simulink model "RTP_V5_Regelung_DKL_Test_P_Regler_Modell_2018a"  (R2020a)
settings: Solver=ode45  StartTime=0.0  StopTime=2  MaxStep=1e-3  RelTol=1e-3  EnableMultiTasking=on
values from neighbouring files (symbols this model uses):
  G_M = cphi    (= 0.03)    [RTP_V5_Regelung_DKL_Test_PIDT1_Regler.m]    (also in RTP_V5_Regelung_DKL_Test_P_Regler.m)
  G_Rueck = cphi    (= 0.03)    [RTP_V5_Regelung_DKL_Test_PIDT1_Regler.m]    (also in RTP_V5_Regelung_DKL_Test_P_Regler.m)
  K = 0.0508    [RTP_V5_Regelung_DKL_Test_PIDT1_Regler.m]    (also in RTP_V5_Regelung_DKL_Test_P_Regler.m = 0.0509)
  n1 = [La/Ra, 1]    [RTP_V5_Regelung_DKL_Test_PIDT1_Regler.m]    (also in RTP_V5_Regelung_DKL_Test_P_Regler.m)
  n3 = [J, 0]    [RTP_V5_Regelung_DKL_Test_PIDT1_Regler.m]    (also in RTP_V5_Regelung_DKL_Test_P_Regler.m)
  n4 = pi    (= 3.14159265359)    [RTP_V5_Regelung_DKL_Test_PIDT1_Regler.m]    (also in RTP_V5_Regelung_DKL_Test_P_Regler.m = 20)
  sat = 1    [RTP_V5_Regelung_DKL_Test_PIDT1_Regler.m]    (also in RTP_V5_Regelung_DKL_Test_P_Regler.m)
  T = 0.004    [RTP_V5_Regelung_DKL_Test_PIDT1_Regler.m]    (also in RTP_V5_Regelung_DKL_Test_P_Regler.m)
  Tn = Tz1 + Tz2 - T    (= 0.129333333333)    [RTP_V5_Regelung_DKL_Test_PIDT1_Regler.m]    (also in RTP_V5_Regelung_DKL_Test_P_Regler.m)
  Tv = Tz1*Tz2 / Tn - T    (= 0.0217731958763)    [RTP_V5_Regelung_DKL_Test_PIDT1_Regler.m]    (also in RTP_V5_Regelung_DKL_Test_P_Regler.m)
  U_mot = 12    [RTP_V5_Regelung_DKL_Test_PIDT1_Regler.m]    (also in RTP_V5_Regelung_DKL_Test_P_Regler.m)
  z1 = 1/Ra    (= 0.285714285714)    [RTP_V5_Regelung_DKL_Test_PIDT1_Regler.m]    (also in RTP_V5_Regelung_DKL_Test_P_Regler.m)
  z3 = 1    [RTP_V5_Regelung_DKL_Test_PIDT1_Regler.m]    (also in RTP_V5_Regelung_DKL_Test_P_Regler.m)
  z4 = i_Getr*180    (= 9)    [RTP_V5_Regelung_DKL_Test_PIDT1_Regler.m]    (also in RTP_V5_Regelung_DKL_Test_P_Regler.m = 57.2957795131)
settings Model: Creator=bruedig  LastModifiedBy=Admin
settings DataIOCC: LimitDataPoints=on  SaveFormat=Array  SignalLoggingSaveFormat=ModelDataLogs  ReturnWorkspaceOutputs=off
settings OptimizationCC: BooleanDataType=off  ExpressionDepthLimit=2147483647  InitFltsAndDblsToZero=on  LifeSpan=inf
settings DebuggingCC: SaveWithParameterizedLinksMsg=none  UnderspecifiedInitializationDetection=Classic  MergeDetectMultiDrivingBlocksExec=none  SignalResolutionControl=TryResolveAllWithWarning  MultiTaskDSMMsg=warning  MultiTaskCondExecSysMsg=none  FcnCallInpInsideContextMsg=warning  StateNameClashWarn=warning  SFUnexpectedBacktrackingDiag=warning  SFNoUnconditionalDefaultTransitionDiag=warning  SFExecutionAtInitializationDiag=none  ArithmeticOperatorsInVariantConditions=warning
settings HardwareCC: ProdBitPerPointer=32  ProdBitPerSizeT=32  ProdBitPerPtrDiffT=32  ProdLargestAtomicFloat=None  ProdIntDivRoundTo=Undefined  ProdEndianess=Unspecified  ProdWordSize=32  ProdHWDeviceType=32-bit Generic  TargetUnknown=on
settings ModelReferenceCC: PropagateSignalLabelsOutOfModel=off
settings SFSimCC: SimUseLocalCustomCode=off  CustomCodeUndefinedFunction=UseInterfaceOnly
settings RTWCC: RTWUseLocalCustomCode=off
settings CodeAppCC: StateflowObjectComments=on
settings GRTTargetCC: TargetFcnLib=ansi_tfl_tmw.mat  TargetLangStandard=C89/C90 (ANSI)  CombineOutputUpdateFcns=off  GRTInterface=on
settings ConfigComp: CovMetricSettings=dw  CovHtmlReporting=on  CovSaveCumulativeToWorkspaceVar=on  CovSaveSingleToWorkspaceVar=on  CovExternalEMLEnable=off

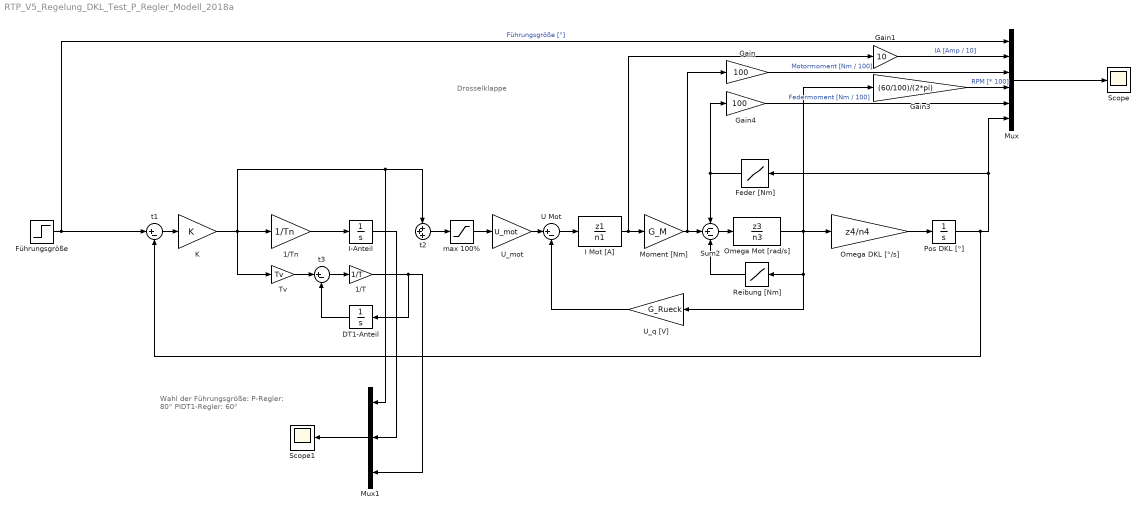
== system RTP_V5_Regelung_DKL_Test_P_Regler_Modell_2018a ==
  note: Wahl der Führungsgröße:
      | P-Regler: 80°
      | PIDT1-Regler: 60°
  note: Drosselklappe
  1/T : Gain  Gain=1/T  SaturateOnIntegerOverflow=on  OutDataTypeStr=Inherit: Same as input  ParamDataTypeStr=Inherit: Same as input
  1/Tn : Gain  Gain=1/Tn  SaturateOnIntegerOverflow=on  OutDataTypeStr=Inherit: Same as input  ParamDataTypeStr=Inherit: Same as input
  DT1-Anteil : Integrator
  Feder [Nm] : Lookup  InputValues="[-0.1,      0,         3.7,     3.8,     90,   90.1]"  Table="[-0.1,   -0.02450,   -0.02430,   0.02430,     0.02916,    0.1]"  SaturateOnIntegerOverflow=on
  Führungsgröße : Step  Time=0  Before=3.7  After=60  SampleTime=0
  Gain : Gain  Gain=100
  Gain1 : Gain  Gain=10
  Gain3 : Gain  Gain=(60/100)/(2*pi)  SaturateOnIntegerOverflow=on  OutDataTypeStr=Inherit: Same as input  ParamDataTypeStr=Inherit: Same as input
  Gain4 : Gain  Gain=100
  I Mot [A] : TransferFcn  Numerator=z1  Denominator=n1
  I-Anteil : Integrator  UpperSaturationLimit=1  LowerSaturationLimit=0
  K : Gain  Gain=K  SaturateOnIntegerOverflow=on  OutDataTypeStr=Inherit: Same as input  ParamDataTypeStr=Inherit: Same as input
  Moment [Nm] : Gain  Gain=G_M  SaturateOnIntegerOverflow=on  OutDataTypeStr=Inherit: Same as input  ParamDataTypeStr=Inherit: Same as input
  Mux : Mux  Inputs=6
  Mux1 : Mux  Inputs=3
  Omega DKL [°/s] : Gain  Gain=z4/n4  SaturateOnIntegerOverflow=on  OutDataTypeStr=Inherit: Same as input  ParamDataTypeStr=Inherit: Same as input
  Omega Mot [rad/s] : TransferFcn  Numerator=z3  Denominator=n3
  Pos DKL [°] : Integrator  InitialCondition=3.7
  Reibung [Nm] : Lookup  InputValues="[-1,              -0.01,           0.01,           1]"  Table="[-0.009,   -0.009,   0.009,   0.009]"  SaturateOnIntegerOverflow=on
  Scope : Scope
  Scope1 : Scope
  Sum2 : Sum  Inputs=-+-  InputSameDT=on  SaturateOnIntegerOverflow=on  OutDataTypeStr=Inherit: Same as first input
  Tv : Gain  Gain=Tv  SaturateOnIntegerOverflow=on  OutDataTypeStr=Inherit: Same as input  ParamDataTypeStr=Inherit: Same as input
  U Mot : Sum  Description=Motorspannung  Inputs=|+-  InputSameDT=on  SaturateOnIntegerOverflow=on  OutDataTypeStr=Inherit: Same as first input
  U_mot : Gain  Gain=U_mot  SaturateOnIntegerOverflow=on  OutDataTypeStr=Inherit: Same as input  ParamDataTypeStr=Inherit: Same as input
  U_q [V] : Gain  Gain=G_Rueck  SaturateOnIntegerOverflow=on  OutDataTypeStr=Inherit: Same as input  ParamDataTypeStr=Inherit: Same as input
  max 100% : Saturate  UpperLimit=sat  LowerLimit=-sat
  t1 : Sum  Description=Motorspannung  Inputs=|+-  InputSameDT=on  SaturateOnIntegerOverflow=on  OutDataTypeStr=Inherit: Same as first input
  t2 : Sum  Description=Motorspannung  Inputs=+++  InputSameDT=on  SaturateOnIntegerOverflow=on  OutDataTypeStr=Inherit: Same as first input
  t3 : Sum  Description=Motorspannung  Inputs=|+-  InputSameDT=on  SaturateOnIntegerOverflow=on  OutDataTypeStr=Inherit: Same as first input
  wires:
  U Mot/1 -> I Mot [A]/1
  Omega Mot [rad/s]/1 -> Omega DKL [°/s]/1, Gain3/1, U_q [V]/1, Reibung [Nm]/1
  Moment [Nm]/1 -> Sum2/2, Gain/1
  Omega DKL [°/s]/1 -> Pos DKL [°]/1
  Sum2/1 -> Omega Mot [rad/s]/1
  I Mot [A]/1 -> Moment [Nm]/1, Gain1/1
  U_q [V]/1 -> U Mot/2
  Mux/1 -> Scope/1
  Gain/1 -> Mux/3  "Motormoment [Nm / 100]"
  Gain1/1 -> Mux/2  "IA [Amp / 10]"
  Führungsgröße/1 -> t1/1, Mux/1  "Führungsgröße [°]"
  Gain3/1 -> Mux/4  "RPM [* 100]"
  Feder [Nm]/1 -> Sum2/1, Gain4/1
  Reibung [Nm]/1 -> Sum2/3
  Gain4/1 -> Mux/5  "Federmoment [Nm / 100]"
  Pos DKL [°]/1 -> Mux/6, Feder [Nm]/1, t1/2
  K/1 -> Tv/1, 1/Tn/1, Mux1/1, t2/1
  t1/1 -> K/1
  U_mot/1 -> U Mot/1
  t2/1 -> max 100%/1
  max 100%/1 -> U_mot/1
  Tv/1 -> t3/1
  t3/1 -> 1/T/1
  1/T/1 -> Mux1/3, DT1-Anteil/1
  1/Tn/1 -> I-Anteil/1
  DT1-Anteil/1 -> t3/2
  I-Anteil/1 -> Mux1/2
  Mux1/1 -> Scope1/1
